simulink model "ExportExample_HIL2"  (Simulink 7.0)
settings: Solver=FixedStepDiscrete  SolverMode=SingleTasking  StartTime=0.0  StopTime=100.0  RelTol=1e-3
InitFcn:
  | %% DSPBuilder Start
  | alt_dspbuilder_update_model(bdroot)
  | %% DSPBuilder End
libraries: allblocks_alteradspbuilder2 x6
settings Model: Creator=lkong  LastModifiedBy=lkong
settings OptimizationCC: InlineInvariantSignals=on
settings DebuggingCC: SaveWithParameterizedLinksMsg=none  SignalResolutionControl=TryResolveAllWithWarning  SolverPrmCheckMsg=none  MultiTaskDSMMsg=warning  MultiTaskCondExecSysMsg=none  StrictBusMsg=None
settings HardwareCC: TargetUnknown=on
settings RTWCC: IncludeERTFirstTime=on
settings GRTTargetCC: TargetFcnLib=ansi_tfl_tmw.mat

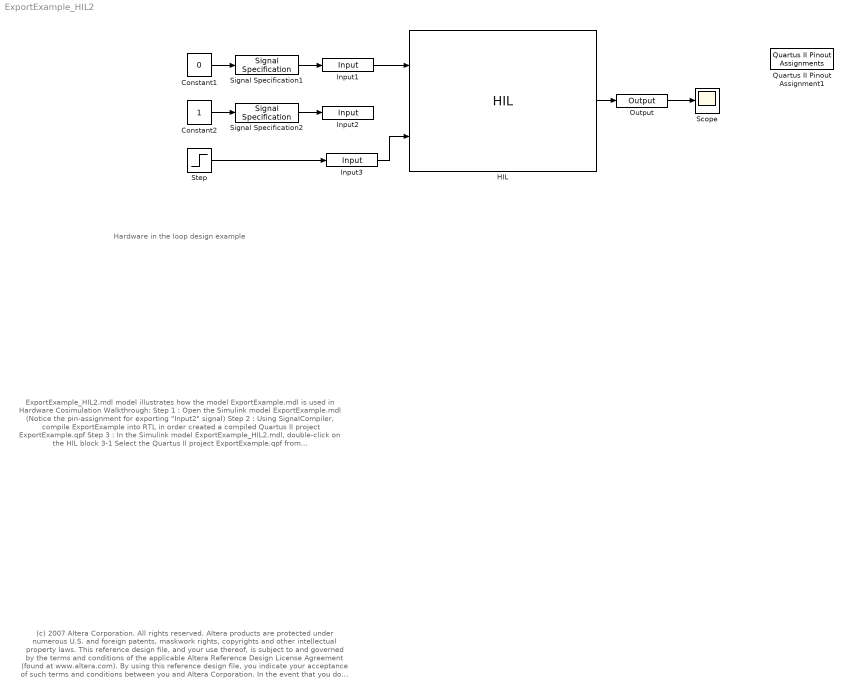
== system ExportExample_HIL2 ==
  note: (c) 2007 Altera Corporation. All rights reserved.  Altera products are protected under numerous U.S. and foreign patents, maskwork rights, copyrights and other intellectual property laws.
      | This reference design file, and your use thereof, is subject to and governed by the terms and conditions of the applicable Altera Reference Design License Agreement (found at www.altera.com).
      | By using this reference design file, you indicate your acceptance of such terms and conditions between you and Altera Corporation.
      | In the event that you do not agree with such terms and conditions, you may not use the reference design file and please promptly destroy any copies you have made.
      | This reference design file being provided on an "as-is" basis and as an accommodation and therefore all warranties, representations or guarantees of any kind (whether express, implied or statutory)
      | including, without limitation, warranties of merchantability, non-infringement, or fitness for a particular purpose, are specifically disclaimed.
      | By making this reference design file available, Altera expressly does not recommend, suggest or require that this reference design file be used in combination with any other product not provided by Altera
  note: Hardware in the loop design example
  note: ExportExample_HIL2.mdl model illustrates how the model ExportExample.mdl is used in Hardware Cosimulation
      |
      | Walkthrough:
      | Step 1 : Open the Simulink model ExportExample.mdl (Notice the pin-assignment for exporting "Input2" signal)
      | Step 2 : Using SignalCompiler, compile ExportExample into RTL in order created a compiled Quartus II project ExportExample.qpf
      | Step 3 : In the Simulink model ExportExample_HIL2.mdl, double-click on the HIL block
      |               3-1 Select the Quartus II project ExportExample.qpf from ExportExample_dspbuilder folder
      |               3-2 Select the Clock and Reset signals
      |               3-3 Change Output to signed
      |               3-4 Select "Input2" and mark it as Export by ticking the Export checkbox
      |               3-5 Select the reset active level to match the settings in the original model
      |               3-6 Click on Goto page 2/2
      |               3-7 Enter the FPGA device value
      |               3-8 Compile with Quartus II
      |               3-9 Scan JTAG ann select the JTAG cable
      |               3-10 Program the FPGA on board
      |               3-11 Close the HIL dialog box
      |
      | Step 4 : Simulate in Simulink
      |               4-1 "Input2" is exported on an FPGA pin connected tp a push-botton SW2 through the pin assignment in the model file,
      |                     press the push-button SW2 on the board while the simulation is running to see the effect on the Scope display
  Constant1 : Constant  Value=0  OutDataType=sfix(16)  OutScaling=2^0
  Constant2 : Constant  OutDataType=sfix(16)  OutScaling=2^0
  HIL : allblocks_alteradspbuilder2/HIL  entityName=ExportExample_HIL2/HIL  inNames=Input1 Input3  inBwls="1  1  1  1  1"  inBwrs="0  0  0  0  0"  inTypes=u u  inDelayed="1  1"  outNames=Output1  outBwls=2  outBwrs=0  outTypes=s  resetNames=aclr  InputCount=5  InputNames=Clock Input1 aclr Input2 Input3  InputWidth="1  1  1  1  1"  InputRepresentation="0  0  0  0  0"  InputExport="2  0  3  1  0"  InputFPP="0  0  0  0  0"  OutputCount=1  OutputNames=Output1  OutputWidth=2  OutputRepresentation=1  OutputExport=0  OutputFPP=0  JtagCable=3  JtagDevice=1  BurstMode=off  BurstLength=1024  FrameMode=off  SOP=1  OutValid=1  QuartusProject=D:\workspace\Documentation\DesignExamples\Tutorials\HIL\ExportExample\ExportExample_dspbuilder\ExportExample.qpf  HilNewConfig=off  ClockPinLocation=K17  ClockPinSource=0  HilDeviceOnBoard=EP2C35F672C6  DR_length=8  dspbuilder_reset=on  SLD_NODE_INFO=9625449  AssertSclrBeforeSimulation=1  SampleTime=-1  dspb_ver=6.1  ResetLevel=Active_High  JtagCableName=USB-Blaster [USB-0]  JtagDeviceName=@1: EP2C35 (0x020B40DD)  ClockNames=Clock
  Input1 : allblocks_alteradspbuilder2/Input  iofile=d:\p4DspbStd81\P4ws\dsp_builder2\Documentation\DesignExamples\Tutorials\HIL\ExportExample\tb_ExportExample_HIL2\ExportExample%5FHIL2_Input1.salt  BusType=Single Bit  bwl=1  bwr=0  SpecifyClock=off  PORTTYPE=Input  externalType=Inferred  allowFloatingPointOverride=on  logOutputs=off
  Input2 : allblocks_alteradspbuilder2/Input  iofile=d:\p4DspbStd81\P4ws\dsp_builder2\Documentation\DesignExamples\Tutorials\HIL\ExportExample\tb_ExportExample_HIL2\ExportExample%5FHIL2_Input2.salt  BusType=Single Bit  bwl=1  bwr=0  SpecifyClock=off  PORTTYPE=Input  externalType=Inferred  allowFloatingPointOverride=on  logOutputs=off
  Input3 : allblocks_alteradspbuilder2/Input  iofile=d:\p4DspbStd81\P4ws\dsp_builder2\Documentation\DesignExamples\Tutorials\HIL\ExportExample\tb_ExportExample_HIL2\ExportExample%5FHIL2_Input3.salt  BusType=Single Bit  bwl=1  bwr=0  SpecifyClock=off  PORTTYPE=Input  externalType=Inferred  allowFloatingPointOverride=on  logOutputs=off
  Output : allblocks_alteradspbuilder2/Output  iofile=d:\p4DspbStd81\P4ws\dsp_builder2\Documentation\DesignExamples\Tutorials\HIL\ExportExample\tb_ExportExample_HIL2\ExportExample%5FHIL2_Output.capture  BusType=Signed Integer  bwl=2  bwr=0  externalType=Inferred  PORTTYPE=Output  allowFloatingPointOverride=on  logOutputs=off
  Quartus II Pinout Assignment1 : allblocks_alteradspbuilder2/Quartus II Pinout Assignments  QuartusIIAssignmentName=Input2  QuartusIIAssignmentValue=Pin_AE14
  Scope : Scope
  Signal Specification1 : SignalSpecification  SampleTime=1  OutDataType=sfix(16)  OutScaling=2^0
  Signal Specification2 : SignalSpecification  SampleTime=1  OutDataType=sfix(16)  OutScaling=2^0
  Step : Step  Time=3  Before=1  After=0  SampleTime=1
  wires:
  Constant2/1 -> Signal Specification2/1
  Constant1/1 -> Signal Specification1/1
  Output/1 -> Scope/1
  HIL/1 -> Output/1
  Input1/1 -> HIL/1
  Signal Specification1/1 -> Input1/1
  Signal Specification2/1 -> Input2/1
  Step/1 -> Input3/1
  Input3/1 -> HIL/2
